simulink model "b6_pfc_rl"  (R2021b)
settings: Solver=FixedStepAuto  StartTime=0.0  StopTime=120.0  FixedStep=0.05  RelTol=1e-3
PreLoadFcn:
  | % Simulation parameters
  | %load exampleMap
  | 
  | % Lidar parameters
  | sensorOffset = [0,0];
  | scanAngles = linspace(-pi/2,pi/2,9)';
  | maxRange = 5;
InitFcn:
  | sampleTime = 0.05;
  | nMedianSize=3;
  | 
  | % Robot parameters
  | wheelRadius = 0.0335;
  | robotRadius = 0.116;
  | 
  | % Lidar parameters
  | sensorOffset = [0,0];
  | scanAngles = linspace(-pi/2,pi/2,9)';
  | maxRange = 5;
  | 
  | %%%%%%
  | ks=1;
  | c_ks=-1;
  | 
  | 
  | 
  | 
  | 
  | 
  | % Lidar parameters
  | sensorOffset = [0,0];
  | scanAngles = linspace(-pi/3,pi/3,20)';%y = linspace(x1,x2,n) 生成 n 个点。这些点的间距为 (x2-x1)/(n-1)。
  | maxRange = 0.4;
  | 
  | %%%%%%
  | ks=1;
  | 
  | 
  | 
  | 
  | 
  | A=0.3;
  | C=1.7;
  | B=(A+C)/2;
  | 
  | wp1=[A,A; B,A;  C,A; C,B;C,C; B,C; A,C;A,B];
  | bainjie2=[-0.5,-0.5;2.5,-0.5;-0.5,2.5;2.5,2.5;]
  | WAY_P=[wp1;wp1;wp1;wp1];
  | Target=[wp1;bainjie2];
  | 
  | %%%%%%%%%%%%%%%%%%%%%%%%%%%%%%%%%%%%%%%
  | Target_robot_4=[A  A]
  | Target_robot_5=[B  A]
  | Target_robot_6=[C  A]
  | 
  | Target_robot_1=[C  C]
  | Target_robot_2=[B  C]
  | Target_robot_3=[A  C]
  | 
  | 
  | %%%%%%%%%%%%%%%%%%%%%%%%%%%%%%%%%%%%
  | 
  | 
  | 
  | 
  | 
  | % paremeters of pure persuit
  | desired_v_robot_1=0.2
  | ... (+42 lines)
undefined symbols (not defined in the file or in its folder): Angular, DiscIntNeverNeededParam, Linear, Pose, Twist
libraries: robotlib x42, dspstat3 x18, mobileRoboticsLib x13, robotmobilelib x6, simulink x2, robotalgslib x1
(part 2 of 3)

== system b6_pfc_rl/controller/Ego Car 4 ==
  pose1 : Inport
  pose2 : Inport  Port=2
  leader_linear_vel : Inport  Port=3
  ego_linear_vel : Inport  Port=4
  ego_omega_vel : Inport  Port=5
  Delay : Delay  DelayLength=1  InitialCondition=0
  Signal Process : MATLAB Function  TreatAsAtomicUnit=on
  obs : Outport
  obs_flag : Outport  Port=2
  wires:
  pose1/1 -> Signal Process/1(pose1)
  Signal Process/1(observation) -> obs/1
  leader_linear_vel/1 -> Signal Process/3(leader_linear_vel)
  ego_omega_vel/1 -> Signal Process/5(ego_omega_vel), Delay/1
  pose2/1 -> Signal Process/2(pose2)
  ego_linear_vel/1 -> Signal Process/4(ego_linear_vel)
  Signal Process/2(obs_flag) -> obs_flag/1
  Delay/1 -> Signal Process/6(last_ego_omega_vel)

== system b6_pfc_rl/controller/Ego Car 5 ==
  pose1 : Inport
  pose2 : Inport  Port=2
  leader_linear_vel : Inport  Port=3
  ego_linear_vel : Inport  Port=4
  ego_omega_vel : Inport  Port=5
  Delay : Delay  DelayLength=1  InitialCondition=0
  Signal Process : MATLAB Function  TreatAsAtomicUnit=on
  obs : Outport
  obs_flag : Outport  Port=2
  wires:
  pose1/1 -> Signal Process/1(pose1)
  Signal Process/1(observation) -> obs/1
  leader_linear_vel/1 -> Signal Process/3(leader_linear_vel)
  ego_omega_vel/1 -> Signal Process/5(ego_omega_vel), Delay/1
  pose2/1 -> Signal Process/2(pose2)
  ego_linear_vel/1 -> Signal Process/4(ego_linear_vel)
  Signal Process/2(obs_flag) -> obs_flag/1
  Delay/1 -> Signal Process/6(last_ego_omega_vel)

== system b6_pfc_rl/controller/Subsystem1 ==
  WayPoints : Inport
  Pose : Inport  Port=2
  0 : Constant  Value=0
  1 : Constant  Value=0
  Adjust Velocities to Avoid Obstacles : Subsystem
  Compute Velocity and Heading for Path following : Subsystem
  Constant1 : Constant  Value=scanAngles
  Outputs1 : Subsystem
  v : Outport
  w : Outport  Port=2
  wires:
  Compute Velocity and Heading for Path following/3(W) -> Adjust Velocities to Avoid Obstacles/2(W), Outputs1/4(W)
  Pose/1 -> Compute Velocity and Heading for Path following/1(CurrentPose)
  Compute Velocity and Heading for Path following/2(V) -> Outputs1/3(V)
  WayPoints/1 -> Compute Velocity and Heading for Path following/2(Waypoints)
  1/1 -> Outputs1/5(CloseToGoal)
  Outputs1/1(v) -> v/1
  Outputs1/2(w) -> w/1
  Adjust Velocities to Avoid Obstacles/1(dW) -> Outputs1/2(dW)
  0/1 -> Outputs1/1(dV)
  Compute Velocity and Heading for Path following/1(TargetDir) -> Adjust Velocities to Avoid Obstacles/1(TargetDir)

== system b6_pfc_rl/controller/signal distribute ==
  In1 : Inport
  Demux5 : Demux  Outputs=12
  Mux{1,3..7} (6 alike) : Mux  Inputs=2
  Mux2 : Mux  Inputs=6
  Out1 : Outport
  wires:
  Mux7/1 -> Mux2/6
  Demux5/4 -> Mux3/2
  Mux1/1 -> Mux2/1
  Demux5/10 -> Mux6/2
  Demux5/7 -> Mux5/1
  Mux5/1 -> Mux2/4
  Mux3/1 -> Mux2/2
  Mux6/1 -> Mux2/5
  Mux4/1 -> Mux2/3
  Demux5/3 -> Mux3/1
  Demux5/8 -> Mux5/2
  Demux5/1 -> Mux1/1
  Demux5/9 -> Mux6/1
  Mux2/1 -> Out1/1
  Demux5/2 -> Mux1/2
  Demux5/11 -> Mux7/1
  Demux5/12 -> Mux7/2
  Demux5/5 -> Mux4/1
  Demux5/6 -> Mux4/2
  In1/1 -> Demux5/1

== system b6_pfc_rl/Subsystem/Car Pose Listener/Subsystem ==
  poseNew : Inport
  poseMsg : Inport  Port=2
  VW_New : Inport  Port=3
  VW_Msg : Inport  Port=4
  DiffSteer Kinematics : Subsystem
      settings: PortSchema="{\"entries\":[{\"content\":{\"sides\":[{\"content\":{\"connectorIds\":[\"In1\",\"In2\"]},\"type\":\"ConnectorPlacement.EquallySpacedRectSide\",\"uuid\":\"0032ed68-1de4-4b1c-b237-9372fedc8a7a\"},{\"content\":{\"connectorIds\":[\"Out1\",\"Out2\",\"Out3\"],\"side\":\"RIGHT\"},\"type\":\"ConnectorPlacement.EquallySpacedRectSide\",\"uuid\":\"d0c861bd-7497-47fe-b183-36da470ee2c6\"},{\"content\":{\"connectorIds\":[\"In3\",\"In4\"],\"side\":\"TOP\"},\"type\":\"ConnectorPlacement.EquallySpacedRectSide\",\"uuid\":\"5b685229-150b-4cb5-b33d-c61d28c4627e\"}]},\"type\":\"ConnectorPlacement.EquallySpacedConnector\",\"uuid\":\"4513c50b-5820-40cb-bb28-cc7c1b1322fe\"}],\"packageUris\":[\"http://schema.mathworks.com/mf0/Connector/R2020b\"],\"version\":\"1.0\"}"
  Median Filter : dspstat3/Median Filter  WindowLength=nMedianSize  SimulateUsing=Interpreted execution
      settings: SourceProductBaseCode=DS
  Median Filter1 : dspstat3/Median Filter  WindowLength=nMedianSize  SimulateUsing=Interpreted execution
      settings: SourceProductBaseCode=DS
  Median Filter2 : dspstat3/Median Filter  WindowLength=nMedianSize  SimulateUsing=Interpreted execution
      settings: SourceProductBaseCode=DS
  Mux7 : Mux  Inputs=3
  Sum : Sum  Inputs=++|
  Sum1 : Sum  Inputs=++|
  sensor2vCar : MATLAB Function  TreatAsAtomicUnit=on
  sensor2vCar4 : MATLAB Function  TreatAsAtomicUnit=on
  pose : Outport
  wires:
  Median Filter2/1 -> Mux7/3
  Median Filter1/1 -> Mux7/2
  Median Filter/1 -> Mux7/1
  sensor2vCar/4(flag) -> DiffSteer Kinematics/3(reset)
  DiffSteer Kinematics/2(y) -> Sum1/2
  sensor2vCar/3(yaw_init) -> DiffSteer Kinematics/4(yaw0)
  sensor2vCar/2(y_init) -> Sum1/1
  sensor2vCar/1(x_init) -> Sum/1
  DiffSteer Kinematics/1(x) -> Sum/2
  VW_New/1 -> sensor2vCar4/1(VW_New)
  Mux7/1 -> pose/1
  Sum/1 -> Median Filter/1
  DiffSteer Kinematics/3(psi) -> Median Filter2/1
  sensor2vCar4/1(V) -> DiffSteer Kinematics/1(u)
  Sum1/1 -> Median Filter1/1
  sensor2vCar4/2(W) -> DiffSteer Kinematics/2(w)
  poseNew/1 -> sensor2vCar/1(poseNew)
  poseMsg/1 -> sensor2vCar/2(poseMsg)
  VW_Msg/1 -> sensor2vCar4/2(VW_Msg)

== system b6_pfc_rl/Subsystem/Car Pose Listener1/Subsystem ==
  poseNew : Inport
  poseMsg : Inport  Port=2
  VW_New : Inport  Port=3
  VW_Msg : Inport  Port=4
  DiffSteer Kinematics : Subsystem
      settings: PortSchema="{\"entries\":[{\"content\":{\"sides\":[{\"content\":{\"connectorIds\":[\"In1\",\"In2\"]},\"type\":\"ConnectorPlacement.EquallySpacedRectSide\",\"uuid\":\"0032ed68-1de4-4b1c-b237-9372fedc8a7a\"},{\"content\":{\"connectorIds\":[\"Out1\",\"Out2\",\"Out3\"],\"side\":\"RIGHT\"},\"type\":\"ConnectorPlacement.EquallySpacedRectSide\",\"uuid\":\"d0c861bd-7497-47fe-b183-36da470ee2c6\"},{\"content\":{\"connectorIds\":[\"In3\",\"In4\"],\"side\":\"TOP\"},\"type\":\"ConnectorPlacement.EquallySpacedRectSide\",\"uuid\":\"5b685229-150b-4cb5-b33d-c61d28c4627e\"}]},\"type\":\"ConnectorPlacement.EquallySpacedConnector\",\"uuid\":\"4513c50b-5820-40cb-bb28-cc7c1b1322fe\"}],\"packageUris\":[\"http://schema.mathworks.com/mf0/Connector/R2020b\"],\"version\":\"1.0\"}"
  Median Filter : dspstat3/Median Filter  WindowLength=nMedianSize  SimulateUsing=Interpreted execution
      settings: SourceProductBaseCode=DS
  Median Filter1 : dspstat3/Median Filter  WindowLength=nMedianSize  SimulateUsing=Interpreted execution
      settings: SourceProductBaseCode=DS
  Median Filter2 : dspstat3/Median Filter  WindowLength=nMedianSize  SimulateUsing=Interpreted execution
      settings: SourceProductBaseCode=DS
  Mux7 : Mux  Inputs=3
  Sum : Sum  Inputs=++|
  Sum1 : Sum  Inputs=++|
  sensor2vCar : MATLAB Function  TreatAsAtomicUnit=on
  sensor2vCar4 : MATLAB Function  TreatAsAtomicUnit=on
  pose : Outport
  wires:
  Median Filter2/1 -> Mux7/3
  Median Filter1/1 -> Mux7/2
  Median Filter/1 -> Mux7/1
  sensor2vCar/4(flag) -> DiffSteer Kinematics/3(reset)
  DiffSteer Kinematics/2(y) -> Sum1/2
  sensor2vCar/3(yaw_init) -> DiffSteer Kinematics/4(yaw0)
  sensor2vCar/2(y_init) -> Sum1/1
  sensor2vCar/1(x_init) -> Sum/1
  DiffSteer Kinematics/1(x) -> Sum/2
  VW_New/1 -> sensor2vCar4/1(VW_New)
  Mux7/1 -> pose/1
  Sum/1 -> Median Filter/1
  DiffSteer Kinematics/3(psi) -> Median Filter2/1
  sensor2vCar4/1(V) -> DiffSteer Kinematics/1(u)
  Sum1/1 -> Median Filter1/1
  sensor2vCar4/2(W) -> DiffSteer Kinematics/2(w)
  poseNew/1 -> sensor2vCar/1(poseNew)
  poseMsg/1 -> sensor2vCar/2(poseMsg)
  VW_Msg/1 -> sensor2vCar4/2(VW_Msg)

== system b6_pfc_rl/Subsystem/Car Pose Listener2/Subsystem ==
  poseNew : Inport
  poseMsg : Inport  Port=2
  VW_New : Inport  Port=3
  VW_Msg : Inport  Port=4
  DiffSteer Kinematics : Subsystem
      settings: PortSchema="{\"entries\":[{\"content\":{\"sides\":[{\"content\":{\"connectorIds\":[\"In1\",\"In2\"]},\"type\":\"ConnectorPlacement.EquallySpacedRectSide\",\"uuid\":\"0032ed68-1de4-4b1c-b237-9372fedc8a7a\"},{\"content\":{\"connectorIds\":[\"Out1\",\"Out2\",\"Out3\"],\"side\":\"RIGHT\"},\"type\":\"ConnectorPlacement.EquallySpacedRectSide\",\"uuid\":\"d0c861bd-7497-47fe-b183-36da470ee2c6\"},{\"content\":{\"connectorIds\":[\"In3\",\"In4\"],\"side\":\"TOP\"},\"type\":\"ConnectorPlacement.EquallySpacedRectSide\",\"uuid\":\"5b685229-150b-4cb5-b33d-c61d28c4627e\"}]},\"type\":\"ConnectorPlacement.EquallySpacedConnector\",\"uuid\":\"4513c50b-5820-40cb-bb28-cc7c1b1322fe\"}],\"packageUris\":[\"http://schema.mathworks.com/mf0/Connector/R2020b\"],\"version\":\"1.0\"}"
  Median Filter : dspstat3/Median Filter  WindowLength=nMedianSize  SimulateUsing=Interpreted execution
      settings: SourceProductBaseCode=DS
  Median Filter1 : dspstat3/Median Filter  WindowLength=nMedianSize  SimulateUsing=Interpreted execution
      settings: SourceProductBaseCode=DS
  Median Filter2 : dspstat3/Median Filter  WindowLength=nMedianSize  SimulateUsing=Interpreted execution
      settings: SourceProductBaseCode=DS
  Mux7 : Mux  Inputs=3
  Sum : Sum  Inputs=++|
  Sum1 : Sum  Inputs=++|
  sensor2vCar : MATLAB Function  TreatAsAtomicUnit=on
  sensor2vCar4 : MATLAB Function  TreatAsAtomicUnit=on
  pose : Outport
  wires:
  Median Filter2/1 -> Mux7/3
  Median Filter1/1 -> Mux7/2
  Median Filter/1 -> Mux7/1
  sensor2vCar/4(flag) -> DiffSteer Kinematics/3(reset)
  DiffSteer Kinematics/2(y) -> Sum1/2
  sensor2vCar/3(yaw_init) -> DiffSteer Kinematics/4(yaw0)
  sensor2vCar/2(y_init) -> Sum1/1
  sensor2vCar/1(x_init) -> Sum/1
  DiffSteer Kinematics/1(x) -> Sum/2
  VW_New/1 -> sensor2vCar4/1(VW_New)
  Mux7/1 -> pose/1
  Sum/1 -> Median Filter/1
  DiffSteer Kinematics/3(psi) -> Median Filter2/1
  sensor2vCar4/1(V) -> DiffSteer Kinematics/1(u)
  Sum1/1 -> Median Filter1/1
  sensor2vCar4/2(W) -> DiffSteer Kinematics/2(w)
  poseNew/1 -> sensor2vCar/1(poseNew)
  poseMsg/1 -> sensor2vCar/2(poseMsg)
  VW_Msg/1 -> sensor2vCar4/2(VW_Msg)

== system b6_pfc_rl/Subsystem/Car Pose Listener3/Subsystem ==
  poseNew : Inport
  poseMsg : Inport  Port=2
  VW_New : Inport  Port=3
  VW_Msg : Inport  Port=4
  DiffSteer Kinematics : Subsystem
      settings: PortSchema="{\"entries\":[{\"content\":{\"sides\":[{\"content\":{\"connectorIds\":[\"In1\",\"In2\"]},\"type\":\"ConnectorPlacement.EquallySpacedRectSide\",\"uuid\":\"0032ed68-1de4-4b1c-b237-9372fedc8a7a\"},{\"content\":{\"connectorIds\":[\"Out1\",\"Out2\",\"Out3\"],\"side\":\"RIGHT\"},\"type\":\"ConnectorPlacement.EquallySpacedRectSide\",\"uuid\":\"d0c861bd-7497-47fe-b183-36da470ee2c6\"},{\"content\":{\"connectorIds\":[\"In3\",\"In4\"],\"side\":\"TOP\"},\"type\":\"ConnectorPlacement.EquallySpacedRectSide\",\"uuid\":\"5b685229-150b-4cb5-b33d-c61d28c4627e\"}]},\"type\":\"ConnectorPlacement.EquallySpacedConnector\",\"uuid\":\"4513c50b-5820-40cb-bb28-cc7c1b1322fe\"}],\"packageUris\":[\"http://schema.mathworks.com/mf0/Connector/R2020b\"],\"version\":\"1.0\"}"
  Median Filter : dspstat3/Median Filter  WindowLength=nMedianSize  SimulateUsing=Interpreted execution
      settings: SourceProductBaseCode=DS
  Median Filter1 : dspstat3/Median Filter  WindowLength=nMedianSize  SimulateUsing=Interpreted execution
      settings: SourceProductBaseCode=DS
  Median Filter2 : dspstat3/Median Filter  WindowLength=nMedianSize  SimulateUsing=Interpreted execution
      settings: SourceProductBaseCode=DS
  Mux7 : Mux  Inputs=3
  Sum : Sum  Inputs=++|
  Sum1 : Sum  Inputs=++|
  sensor2vCar : MATLAB Function  TreatAsAtomicUnit=on
  sensor2vCar4 : MATLAB Function  TreatAsAtomicUnit=on
  pose : Outport
  wires:
  Median Filter2/1 -> Mux7/3
  Median Filter1/1 -> Mux7/2
  Median Filter/1 -> Mux7/1
  sensor2vCar/4(flag) -> DiffSteer Kinematics/3(reset)
  DiffSteer Kinematics/2(y) -> Sum1/2
  sensor2vCar/3(yaw_init) -> DiffSteer Kinematics/4(yaw0)
  sensor2vCar/2(y_init) -> Sum1/1
  sensor2vCar/1(x_init) -> Sum/1
  DiffSteer Kinematics/1(x) -> Sum/2
  VW_New/1 -> sensor2vCar4/1(VW_New)
  Mux7/1 -> pose/1
  Sum/1 -> Median Filter/1
  DiffSteer Kinematics/3(psi) -> Median Filter2/1
  sensor2vCar4/1(V) -> DiffSteer Kinematics/1(u)
  Sum1/1 -> Median Filter1/1
  sensor2vCar4/2(W) -> DiffSteer Kinematics/2(w)
  poseNew/1 -> sensor2vCar/1(poseNew)
  poseMsg/1 -> sensor2vCar/2(poseMsg)
  VW_Msg/1 -> sensor2vCar4/2(VW_Msg)

== system b6_pfc_rl/Subsystem/Car Pose Listener4/Subsystem ==
  poseNew : Inport
  poseMsg : Inport  Port=2
  VW_New : Inport  Port=3
  VW_Msg : Inport  Port=4
  DiffSteer Kinematics : Subsystem
      settings: PortSchema="{\"entries\":[{\"content\":{\"sides\":[{\"content\":{\"connectorIds\":[\"In1\",\"In2\"]},\"type\":\"ConnectorPlacement.EquallySpacedRectSide\",\"uuid\":\"0032ed68-1de4-4b1c-b237-9372fedc8a7a\"},{\"content\":{\"connectorIds\":[\"Out1\",\"Out2\",\"Out3\"],\"side\":\"RIGHT\"},\"type\":\"ConnectorPlacement.EquallySpacedRectSide\",\"uuid\":\"d0c861bd-7497-47fe-b183-36da470ee2c6\"},{\"content\":{\"connectorIds\":[\"In3\",\"In4\"],\"side\":\"TOP\"},\"type\":\"ConnectorPlacement.EquallySpacedRectSide\",\"uuid\":\"5b685229-150b-4cb5-b33d-c61d28c4627e\"}]},\"type\":\"ConnectorPlacement.EquallySpacedConnector\",\"uuid\":\"4513c50b-5820-40cb-bb28-cc7c1b1322fe\"}],\"packageUris\":[\"http://schema.mathworks.com/mf0/Connector/R2020b\"],\"version\":\"1.0\"}"
  Median Filter : dspstat3/Median Filter  WindowLength=nMedianSize  SimulateUsing=Interpreted execution
      settings: SourceProductBaseCode=DS
  Median Filter1 : dspstat3/Median Filter  WindowLength=nMedianSize  SimulateUsing=Interpreted execution
      settings: SourceProductBaseCode=DS
  Median Filter2 : dspstat3/Median Filter  WindowLength=nMedianSize  SimulateUsing=Interpreted execution
      settings: SourceProductBaseCode=DS
  Mux7 : Mux  Inputs=3
  Sum : Sum  Inputs=++|
  Sum1 : Sum  Inputs=++|
  sensor2vCar : MATLAB Function  TreatAsAtomicUnit=on
  sensor2vCar4 : MATLAB Function  TreatAsAtomicUnit=on
  pose : Outport
  wires:
  Median Filter2/1 -> Mux7/3
  Median Filter1/1 -> Mux7/2
  Median Filter/1 -> Mux7/1
  sensor2vCar/4(flag) -> DiffSteer Kinematics/3(reset)
  DiffSteer Kinematics/2(y) -> Sum1/2
  sensor2vCar/3(yaw_init) -> DiffSteer Kinematics/4(yaw0)
  sensor2vCar/2(y_init) -> Sum1/1
  sensor2vCar/1(x_init) -> Sum/1
  DiffSteer Kinematics/1(x) -> Sum/2
  VW_New/1 -> sensor2vCar4/1(VW_New)
  Mux7/1 -> pose/1
  Sum/1 -> Median Filter/1
  DiffSteer Kinematics/3(psi) -> Median Filter2/1
  sensor2vCar4/1(V) -> DiffSteer Kinematics/1(u)
  Sum1/1 -> Median Filter1/1
  sensor2vCar4/2(W) -> DiffSteer Kinematics/2(w)
  poseNew/1 -> sensor2vCar/1(poseNew)
  poseMsg/1 -> sensor2vCar/2(poseMsg)
  VW_Msg/1 -> sensor2vCar4/2(VW_Msg)

== system b6_pfc_rl/Subsystem/Car Pose Listener5/Subsystem ==
  poseNew : Inport
  poseMsg : Inport  Port=2
  VW_New : Inport  Port=3
  VW_Msg : Inport  Port=4
  DiffSteer Kinematics : Subsystem
      settings: PortSchema="{\"entries\":[{\"content\":{\"sides\":[{\"content\":{\"connectorIds\":[\"In1\",\"In2\"]},\"type\":\"ConnectorPlacement.EquallySpacedRectSide\",\"uuid\":\"0032ed68-1de4-4b1c-b237-9372fedc8a7a\"},{\"content\":{\"connectorIds\":[\"Out1\",\"Out2\",\"Out3\"],\"side\":\"RIGHT\"},\"type\":\"ConnectorPlacement.EquallySpacedRectSide\",\"uuid\":\"d0c861bd-7497-47fe-b183-36da470ee2c6\"},{\"content\":{\"connectorIds\":[\"In3\",\"In4\"],\"side\":\"TOP\"},\"type\":\"ConnectorPlacement.EquallySpacedRectSide\",\"uuid\":\"5b685229-150b-4cb5-b33d-c61d28c4627e\"}]},\"type\":\"ConnectorPlacement.EquallySpacedConnector\",\"uuid\":\"4513c50b-5820-40cb-bb28-cc7c1b1322fe\"}],\"packageUris\":[\"http://schema.mathworks.com/mf0/Connector/R2020b\"],\"version\":\"1.0\"}"
  Median Filter : dspstat3/Median Filter  WindowLength=nMedianSize  SimulateUsing=Interpreted execution
      settings: SourceProductBaseCode=DS
  Median Filter1 : dspstat3/Median Filter  WindowLength=nMedianSize  SimulateUsing=Interpreted execution
      settings: SourceProductBaseCode=DS
  Median Filter2 : dspstat3/Median Filter  WindowLength=nMedianSize  SimulateUsing=Interpreted execution
      settings: SourceProductBaseCode=DS
  Mux7 : Mux  Inputs=3
  Sum : Sum  Inputs=++|
  Sum1 : Sum  Inputs=++|
  sensor2vCar : MATLAB Function  TreatAsAtomicUnit=on
  sensor2vCar4 : MATLAB Function  TreatAsAtomicUnit=on
  pose : Outport
  wires:
  Median Filter2/1 -> Mux7/3
  Median Filter1/1 -> Mux7/2
  Median Filter/1 -> Mux7/1
  sensor2vCar/4(flag) -> DiffSteer Kinematics/3(reset)
  DiffSteer Kinematics/2(y) -> Sum1/2
  sensor2vCar/3(yaw_init) -> DiffSteer Kinematics/4(yaw0)
  sensor2vCar/2(y_init) -> Sum1/1
  sensor2vCar/1(x_init) -> Sum/1
  DiffSteer Kinematics/1(x) -> Sum/2
  VW_New/1 -> sensor2vCar4/1(VW_New)
  Mux7/1 -> pose/1
  Sum/1 -> Median Filter/1
  DiffSteer Kinematics/3(psi) -> Median Filter2/1
  sensor2vCar4/1(V) -> DiffSteer Kinematics/1(u)
  Sum1/1 -> Median Filter1/1
  sensor2vCar4/2(W) -> DiffSteer Kinematics/2(w)
  poseNew/1 -> sensor2vCar/1(poseNew)
  poseMsg/1 -> sensor2vCar/2(poseMsg)
  VW_Msg/1 -> sensor2vCar4/2(VW_Msg)

== system b6_pfc_rl/controller/Subsystem1/Adjust Velocities to Avoid Obstacles ==
  TargetDir : Inport
  W : Inport  Port=2
  Path Following : Subsystem  TreatAsAtomicUnit=on
  dW : Outport  VectorParamsAs1DForOutWhenUnconnected=off
  wires:
  Path Following/1(dW) -> dW/1
  W/1 -> Path Following/2(AngularVelocity)
  TargetDir/1 -> Path Following/1(SteeringDirection)

== system b6_pfc_rl/controller/Subsystem1/Compute Velocity and Heading for Path following ==
  note: Check If Close To Goal
  CurrentPose : Inport
  Waypoints : Inport  Port=2
  " Extract Goal" : MATLAB Function  TreatAsAtomicUnit=on
  Dot Product : DotProduct  InputSameDT=on  OutDataTypeStr=Inherit: Inherit via internal rule
  GoalRadius : Constant  Value=0.1
  Pure Pursuit : robotalgslib/Pure Pursuit  DesiredLinearVelocity=desired_v_robot_1  MaxAngularVelocity=desired_w_robot_1  LookaheadDistance=desired_lookahead_robot_1  TargetDirPort=on  SimulateUsing=Code generation
  Relational Operator : RelationalOperator  Operator=<=  OutDataTypeStr=boolean  RndMeth=Simplest
  Selector : Selector  InputPortWidth=3  IndexOptions=Index vector (dialog)  Indices=[1 2]  OutputSizes=1
  Sqrt : Sqrt  SaturateOnIntegerOverflow=on
  Subtract : Sum  Inputs=+-
  TargetDir : Outport  VectorParamsAs1DForOutWhenUnconnected=off
  V : Outport  Port=2  VectorParamsAs1DForOutWhenUnconnected=off
  W : Outport  Port=3  VectorParamsAs1DForOutWhenUnconnected=off
  CloseToGoal : Outport  Port=4  VectorParamsAs1DForOutWhenUnconnected=off
  wires:
  Pure Pursuit/3 -> TargetDir/1
  Pure Pursuit/2 -> W/1
  Pure Pursuit/1 -> V/1
  " Extract Goal"/1(Goal) -> Subtract/2
  Waypoints/1 -> " Extract Goal"/1(Waypoints), Pure Pursuit/2
  CurrentPose/1 -> Selector/1, Pure Pursuit/1
  Relational Operator/1 -> CloseToGoal/1
  GoalRadius/1 -> Relational Operator/2
  Selector/1 -> Subtract/1
  Dot Product/1 -> Sqrt/1
  Sqrt/1 -> Relational Operator/1
  Subtract/1 -> Dot Product/1, Dot Product/2

== system b6_pfc_rl/controller/Subsystem1/Outputs1 ==
  dV : Inport
  dW : Inport  Port=2
  V : Inport  Port=3
  W : Inport  Port=4
  CloseToGoal : Inport  Port=5
  Add : Sum
  Add1 : Sum
  Logical Operator : Logic  Operator=NOT  AllPortsSameDT=off  OutDataTypeStr=boolean
  Product : Product
  Product1 : Product
  v : Outport
  w : Outport  Port=2
  wires:
  V/1 -> Add/2
  W/1 -> Add1/2
  dV/1 -> Add/1
  dW/1 -> Add1/1
  CloseToGoal/1 -> Logical Operator/1
  Add/1 -> Product/1
  Add1/1 -> Product1/1
  Product1/1 -> w/1
  Product/1 -> v/1
  Logical Operator/1 -> Product1/2, Product/2

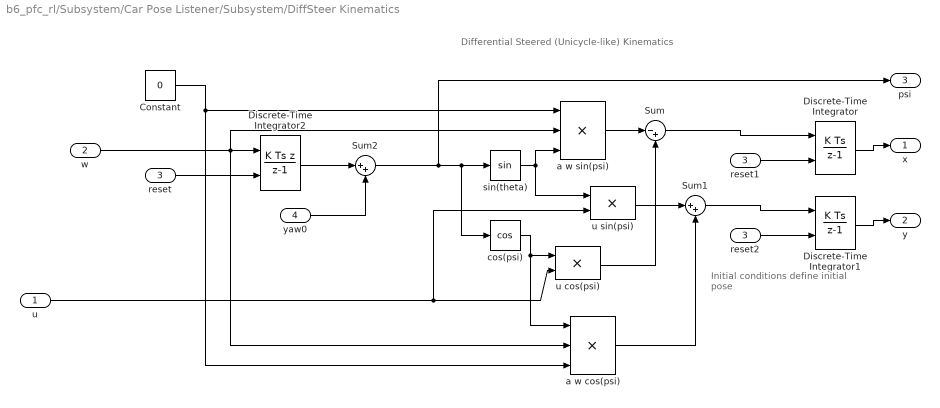
== system b6_pfc_rl/Subsystem/Car Pose Listener/Subsystem/DiffSteer Kinematics ==
  note: Initial conditions define
      | initial pose
  note: Differential Steered (Unicycle-like) Kinematics
  u : Inport
  w : Inport  Port=2
  reset : Inport  Port=3
  yaw0 : Inport  Port=4
  Constant : Constant  Value=0
  Discrete-Time Integrator : DiscreteIntegrator  ExternalReset=falling  SampleTime=-1  ICPrevOutput=DiscIntNeverNeededParam  ICPrevScaledInput=DiscIntNeverNeededParam
  Discrete-Time Integrator1 : DiscreteIntegrator  ExternalReset=falling  SampleTime=-1  ICPrevOutput=DiscIntNeverNeededParam  ICPrevScaledInput=DiscIntNeverNeededParam
  Discrete-Time Integrator2 : DiscreteIntegrator  IntegratorMethod=Integration: Backward Euler  ExternalReset=falling  SampleTime=-1  ICPrevOutput=DiscIntNeverNeededParam  ICPrevScaledInput=DiscIntNeverNeededParam
  Sum : Sum  Inputs=|-+  SaturateOnIntegerOverflow=on
  Sum1 : Sum  Inputs=|++  SaturateOnIntegerOverflow=on
  Sum2 : Sum  Inputs=|++
  a w cos(psi) : Product  Inputs=3  SaturateOnIntegerOverflow=on  OutDataTypeStr=Inherit: Same as first input
  a w sin(psi) : Product  Inputs=3  SaturateOnIntegerOverflow=on  OutDataTypeStr=Inherit: Same as first input
  cos(psi) : Trigonometry  Operator=cos
  reset1 : InportShadow  Port=3
  reset2 : InportShadow  Port=3
  sin(theta) : Trigonometry
  u cos(psi) : Product  SaturateOnIntegerOverflow=on  OutDataTypeStr=Inherit: Same as first input
  u sin(psi) : Product  SaturateOnIntegerOverflow=on  OutDataTypeStr=Inherit: Same as first input
  x : Outport
  y : Outport  Port=2
  psi : Outport  Port=3
  wires:
  yaw0/1 -> Sum2/2
  reset2/1 -> Discrete-Time Integrator1/2
  reset1/1 -> Discrete-Time Integrator/2
  reset/1 -> Discrete-Time Integrator2/2
  u sin(psi)/1 -> Sum1/1
  cos(psi)/1 -> u cos(psi)/1, a w cos(psi)/1
  w/1 -> a w cos(psi)/2, a w sin(psi)/2, Discrete-Time Integrator2/1
  Constant/1 -> a w sin(psi)/1, a w cos(psi)/3
  Discrete-Time Integrator/1 -> x/1
  Sum/1 -> Discrete-Time Integrator/1
  sin(theta)/1 -> a w sin(psi)/3, u sin(psi)/1
  a w cos(psi)/1 -> Sum1/2
  Sum2/1 -> psi/1, sin(theta)/1, cos(psi)/1
  u cos(psi)/1 -> Sum/2
  u/1 -> u sin(psi)/2, u cos(psi)/2
  a w sin(psi)/1 -> Sum/1
  Sum1/1 -> Discrete-Time Integrator1/1
  Discrete-Time Integrator1/1 -> y/1
  Discrete-Time Integrator2/1 -> Sum2/1

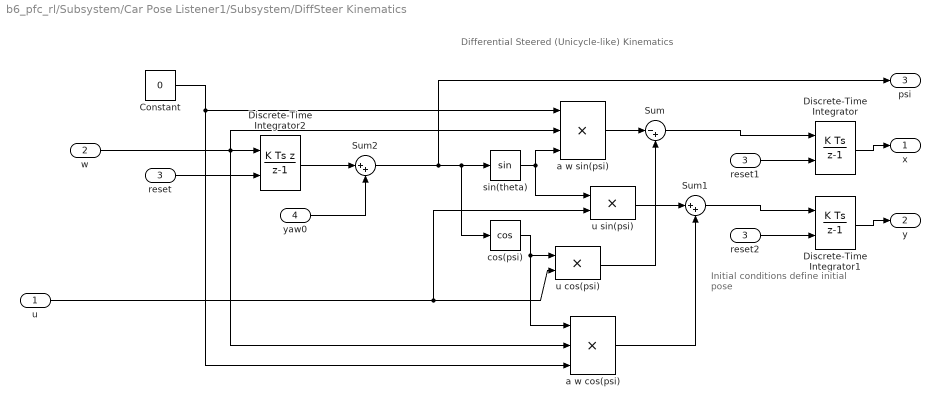
== system b6_pfc_rl/Subsystem/Car Pose Listener1/Subsystem/DiffSteer Kinematics ==
  note: Initial conditions define
      | initial pose
  note: Differential Steered (Unicycle-like) Kinematics
  u : Inport
  w : Inport  Port=2
  reset : Inport  Port=3
  yaw0 : Inport  Port=4
  Constant : Constant  Value=0
  Discrete-Time Integrator : DiscreteIntegrator  ExternalReset=falling  SampleTime=-1  ICPrevOutput=DiscIntNeverNeededParam  ICPrevScaledInput=DiscIntNeverNeededParam
  Discrete-Time Integrator1 : DiscreteIntegrator  ExternalReset=falling  SampleTime=-1  ICPrevOutput=DiscIntNeverNeededParam  ICPrevScaledInput=DiscIntNeverNeededParam
  Discrete-Time Integrator2 : DiscreteIntegrator  IntegratorMethod=Integration: Backward Euler  ExternalReset=falling  SampleTime=-1  ICPrevOutput=DiscIntNeverNeededParam  ICPrevScaledInput=DiscIntNeverNeededParam
  Sum : Sum  Inputs=|-+  SaturateOnIntegerOverflow=on
  Sum1 : Sum  Inputs=|++  SaturateOnIntegerOverflow=on
  Sum2 : Sum  Inputs=|++
  a w cos(psi) : Product  Inputs=3  SaturateOnIntegerOverflow=on  OutDataTypeStr=Inherit: Same as first input
  a w sin(psi) : Product  Inputs=3  SaturateOnIntegerOverflow=on  OutDataTypeStr=Inherit: Same as first input
  cos(psi) : Trigonometry  Operator=cos
  reset1 : InportShadow  Port=3
  reset2 : InportShadow  Port=3
  sin(theta) : Trigonometry
  u cos(psi) : Product  SaturateOnIntegerOverflow=on  OutDataTypeStr=Inherit: Same as first input
  u sin(psi) : Product  SaturateOnIntegerOverflow=on  OutDataTypeStr=Inherit: Same as first input
  x : Outport
  y : Outport  Port=2
  psi : Outport  Port=3
  wires:
  yaw0/1 -> Sum2/2
  reset2/1 -> Discrete-Time Integrator1/2
  reset1/1 -> Discrete-Time Integrator/2
  reset/1 -> Discrete-Time Integrator2/2
  u sin(psi)/1 -> Sum1/1
  cos(psi)/1 -> u cos(psi)/1, a w cos(psi)/1
  w/1 -> a w cos(psi)/2, a w sin(psi)/2, Discrete-Time Integrator2/1
  Constant/1 -> a w sin(psi)/1, a w cos(psi)/3
  Discrete-Time Integrator/1 -> x/1
  Sum/1 -> Discrete-Time Integrator/1
  sin(theta)/1 -> a w sin(psi)/3, u sin(psi)/1
  a w cos(psi)/1 -> Sum1/2
  Sum2/1 -> psi/1, sin(theta)/1, cos(psi)/1
  u cos(psi)/1 -> Sum/2
  u/1 -> u sin(psi)/2, u cos(psi)/2
  a w sin(psi)/1 -> Sum/1
  Sum1/1 -> Discrete-Time Integrator1/1
  Discrete-Time Integrator1/1 -> y/1
  Discrete-Time Integrator2/1 -> Sum2/1

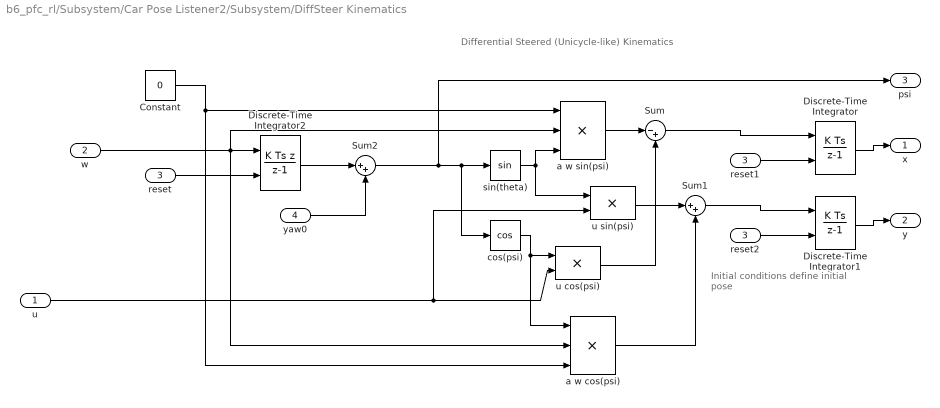
== system b6_pfc_rl/Subsystem/Car Pose Listener2/Subsystem/DiffSteer Kinematics ==
  note: Initial conditions define
      | initial pose
  note: Differential Steered (Unicycle-like) Kinematics
  u : Inport
  w : Inport  Port=2
  reset : Inport  Port=3
  yaw0 : Inport  Port=4
  Constant : Constant  Value=0
  Discrete-Time Integrator : DiscreteIntegrator  ExternalReset=falling  SampleTime=-1  ICPrevOutput=DiscIntNeverNeededParam  ICPrevScaledInput=DiscIntNeverNeededParam
  Discrete-Time Integrator1 : DiscreteIntegrator  ExternalReset=falling  SampleTime=-1  ICPrevOutput=DiscIntNeverNeededParam  ICPrevScaledInput=DiscIntNeverNeededParam
  Discrete-Time Integrator2 : DiscreteIntegrator  IntegratorMethod=Integration: Backward Euler  ExternalReset=falling  SampleTime=-1  ICPrevOutput=DiscIntNeverNeededParam  ICPrevScaledInput=DiscIntNeverNeededParam
  Sum : Sum  Inputs=|-+  SaturateOnIntegerOverflow=on
  Sum1 : Sum  Inputs=|++  SaturateOnIntegerOverflow=on
  Sum2 : Sum  Inputs=|++
  a w cos(psi) : Product  Inputs=3  SaturateOnIntegerOverflow=on  OutDataTypeStr=Inherit: Same as first input
  a w sin(psi) : Product  Inputs=3  SaturateOnIntegerOverflow=on  OutDataTypeStr=Inherit: Same as first input
  cos(psi) : Trigonometry  Operator=cos
  reset1 : InportShadow  Port=3
  reset2 : InportShadow  Port=3
  sin(theta) : Trigonometry
  u cos(psi) : Product  SaturateOnIntegerOverflow=on  OutDataTypeStr=Inherit: Same as first input
  u sin(psi) : Product  SaturateOnIntegerOverflow=on  OutDataTypeStr=Inherit: Same as first input
  x : Outport
  y : Outport  Port=2
  psi : Outport  Port=3
  wires:
  yaw0/1 -> Sum2/2
  reset2/1 -> Discrete-Time Integrator1/2
  reset1/1 -> Discrete-Time Integrator/2
  reset/1 -> Discrete-Time Integrator2/2
  u sin(psi)/1 -> Sum1/1
  cos(psi)/1 -> u cos(psi)/1, a w cos(psi)/1
  w/1 -> a w cos(psi)/2, a w sin(psi)/2, Discrete-Time Integrator2/1
  Constant/1 -> a w sin(psi)/1, a w cos(psi)/3
  Discrete-Time Integrator/1 -> x/1
  Sum/1 -> Discrete-Time Integrator/1
  sin(theta)/1 -> a w sin(psi)/3, u sin(psi)/1
  a w cos(psi)/1 -> Sum1/2
  Sum2/1 -> psi/1, sin(theta)/1, cos(psi)/1
  u cos(psi)/1 -> Sum/2
  u/1 -> u sin(psi)/2, u cos(psi)/2
  a w sin(psi)/1 -> Sum/1
  Sum1/1 -> Discrete-Time Integrator1/1
  Discrete-Time Integrator1/1 -> y/1
  Discrete-Time Integrator2/1 -> Sum2/1

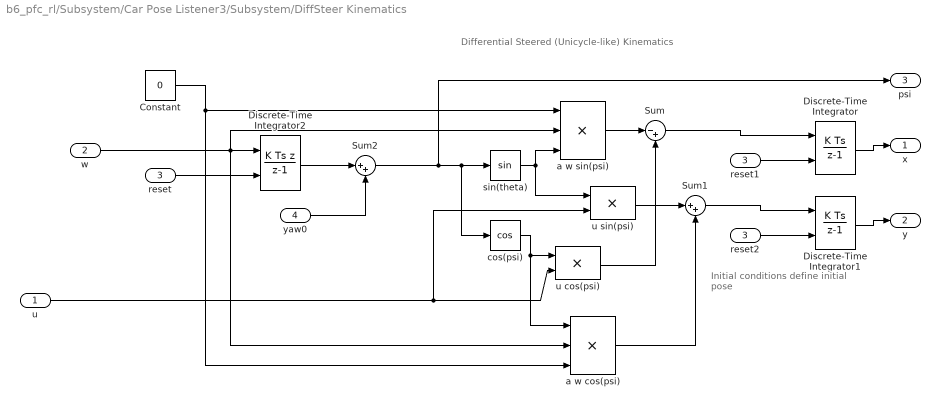
== system b6_pfc_rl/Subsystem/Car Pose Listener3/Subsystem/DiffSteer Kinematics ==
  note: Initial conditions define
      | initial pose
  note: Differential Steered (Unicycle-like) Kinematics
  u : Inport
  w : Inport  Port=2
  reset : Inport  Port=3
  yaw0 : Inport  Port=4
  Constant : Constant  Value=0
  Discrete-Time Integrator : DiscreteIntegrator  ExternalReset=falling  SampleTime=-1  ICPrevOutput=DiscIntNeverNeededParam  ICPrevScaledInput=DiscIntNeverNeededParam
  Discrete-Time Integrator1 : DiscreteIntegrator  ExternalReset=falling  SampleTime=-1  ICPrevOutput=DiscIntNeverNeededParam  ICPrevScaledInput=DiscIntNeverNeededParam
  Discrete-Time Integrator2 : DiscreteIntegrator  IntegratorMethod=Integration: Backward Euler  ExternalReset=falling  SampleTime=-1  ICPrevOutput=DiscIntNeverNeededParam  ICPrevScaledInput=DiscIntNeverNeededParam
  Sum : Sum  Inputs=|-+  SaturateOnIntegerOverflow=on
  Sum1 : Sum  Inputs=|++  SaturateOnIntegerOverflow=on
  Sum2 : Sum  Inputs=|++
  a w cos(psi) : Product  Inputs=3  SaturateOnIntegerOverflow=on  OutDataTypeStr=Inherit: Same as first input
  a w sin(psi) : Product  Inputs=3  SaturateOnIntegerOverflow=on  OutDataTypeStr=Inherit: Same as first input
  cos(psi) : Trigonometry  Operator=cos
  reset1 : InportShadow  Port=3
  reset2 : InportShadow  Port=3
  sin(theta) : Trigonometry
  u cos(psi) : Product  SaturateOnIntegerOverflow=on  OutDataTypeStr=Inherit: Same as first input
  u sin(psi) : Product  SaturateOnIntegerOverflow=on  OutDataTypeStr=Inherit: Same as first input
  x : Outport
  y : Outport  Port=2
  psi : Outport  Port=3
  wires:
  yaw0/1 -> Sum2/2
  reset2/1 -> Discrete-Time Integrator1/2
  reset1/1 -> Discrete-Time Integrator/2
  reset/1 -> Discrete-Time Integrator2/2
  u sin(psi)/1 -> Sum1/1
  cos(psi)/1 -> u cos(psi)/1, a w cos(psi)/1
  w/1 -> a w cos(psi)/2, a w sin(psi)/2, Discrete-Time Integrator2/1
  Constant/1 -> a w sin(psi)/1, a w cos(psi)/3
  Discrete-Time Integrator/1 -> x/1
  Sum/1 -> Discrete-Time Integrator/1
  sin(theta)/1 -> a w sin(psi)/3, u sin(psi)/1
  a w cos(psi)/1 -> Sum1/2
  Sum2/1 -> psi/1, sin(theta)/1, cos(psi)/1
  u cos(psi)/1 -> Sum/2
  u/1 -> u sin(psi)/2, u cos(psi)/2
  a w sin(psi)/1 -> Sum/1
  Sum1/1 -> Discrete-Time Integrator1/1
  Discrete-Time Integrator1/1 -> y/1
  Discrete-Time Integrator2/1 -> Sum2/1

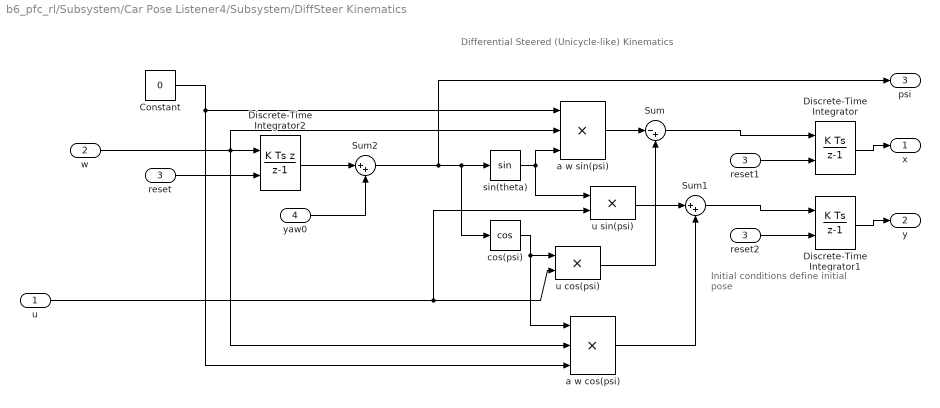
== system b6_pfc_rl/Subsystem/Car Pose Listener4/Subsystem/DiffSteer Kinematics ==
  note: Initial conditions define
      | initial pose
  note: Differential Steered (Unicycle-like) Kinematics
  u : Inport
  w : Inport  Port=2
  reset : Inport  Port=3
  yaw0 : Inport  Port=4
  Constant : Constant  Value=0
  Discrete-Time Integrator : DiscreteIntegrator  ExternalReset=falling  SampleTime=-1  ICPrevOutput=DiscIntNeverNeededParam  ICPrevScaledInput=DiscIntNeverNeededParam
  Discrete-Time Integrator1 : DiscreteIntegrator  ExternalReset=falling  SampleTime=-1  ICPrevOutput=DiscIntNeverNeededParam  ICPrevScaledInput=DiscIntNeverNeededParam
  Discrete-Time Integrator2 : DiscreteIntegrator  IntegratorMethod=Integration: Backward Euler  ExternalReset=falling  SampleTime=-1  ICPrevOutput=DiscIntNeverNeededParam  ICPrevScaledInput=DiscIntNeverNeededParam
  Sum : Sum  Inputs=|-+  SaturateOnIntegerOverflow=on
  Sum1 : Sum  Inputs=|++  SaturateOnIntegerOverflow=on
  Sum2 : Sum  Inputs=|++
  a w cos(psi) : Product  Inputs=3  SaturateOnIntegerOverflow=on  OutDataTypeStr=Inherit: Same as first input
  a w sin(psi) : Product  Inputs=3  SaturateOnIntegerOverflow=on  OutDataTypeStr=Inherit: Same as first input
  cos(psi) : Trigonometry  Operator=cos
  reset1 : InportShadow  Port=3
  reset2 : InportShadow  Port=3
  sin(theta) : Trigonometry
  u cos(psi) : Product  SaturateOnIntegerOverflow=on  OutDataTypeStr=Inherit: Same as first input
  u sin(psi) : Product  SaturateOnIntegerOverflow=on  OutDataTypeStr=Inherit: Same as first input
  x : Outport
  y : Outport  Port=2
  psi : Outport  Port=3
  wires:
  yaw0/1 -> Sum2/2
  reset2/1 -> Discrete-Time Integrator1/2
  reset1/1 -> Discrete-Time Integrator/2
  reset/1 -> Discrete-Time Integrator2/2
  u sin(psi)/1 -> Sum1/1
  cos(psi)/1 -> u cos(psi)/1, a w cos(psi)/1
  w/1 -> a w cos(psi)/2, a w sin(psi)/2, Discrete-Time Integrator2/1
  Constant/1 -> a w sin(psi)/1, a w cos(psi)/3
  Discrete-Time Integrator/1 -> x/1
  Sum/1 -> Discrete-Time Integrator/1
  sin(theta)/1 -> a w sin(psi)/3, u sin(psi)/1
  a w cos(psi)/1 -> Sum1/2
  Sum2/1 -> psi/1, sin(theta)/1, cos(psi)/1
  u cos(psi)/1 -> Sum/2
  u/1 -> u sin(psi)/2, u cos(psi)/2
  a w sin(psi)/1 -> Sum/1
  Sum1/1 -> Discrete-Time Integrator1/1
  Discrete-Time Integrator1/1 -> y/1
  Discrete-Time Integrator2/1 -> Sum2/1

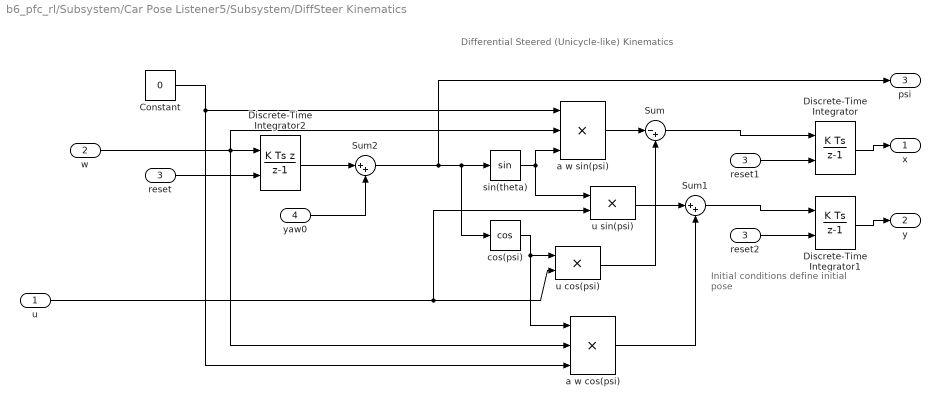
== system b6_pfc_rl/Subsystem/Car Pose Listener5/Subsystem/DiffSteer Kinematics ==
  note: Initial conditions define
      | initial pose
  note: Differential Steered (Unicycle-like) Kinematics
  u : Inport
  w : Inport  Port=2
  reset : Inport  Port=3
  yaw0 : Inport  Port=4
  Constant : Constant  Value=0
  Discrete-Time Integrator : DiscreteIntegrator  ExternalReset=falling  SampleTime=-1  ICPrevOutput=DiscIntNeverNeededParam  ICPrevScaledInput=DiscIntNeverNeededParam
  Discrete-Time Integrator1 : DiscreteIntegrator  ExternalReset=falling  SampleTime=-1  ICPrevOutput=DiscIntNeverNeededParam  ICPrevScaledInput=DiscIntNeverNeededParam
  Discrete-Time Integrator2 : DiscreteIntegrator  IntegratorMethod=Integration: Backward Euler  ExternalReset=falling  SampleTime=-1  ICPrevOutput=DiscIntNeverNeededParam  ICPrevScaledInput=DiscIntNeverNeededParam
  Sum : Sum  Inputs=|-+  SaturateOnIntegerOverflow=on
  Sum1 : Sum  Inputs=|++  SaturateOnIntegerOverflow=on
  Sum2 : Sum  Inputs=|++
  a w cos(psi) : Product  Inputs=3  SaturateOnIntegerOverflow=on  OutDataTypeStr=Inherit: Same as first input
  a w sin(psi) : Product  Inputs=3  SaturateOnIntegerOverflow=on  OutDataTypeStr=Inherit: Same as first input
  cos(psi) : Trigonometry  Operator=cos
  reset1 : InportShadow  Port=3
  reset2 : InportShadow  Port=3
  sin(theta) : Trigonometry
  u cos(psi) : Product  SaturateOnIntegerOverflow=on  OutDataTypeStr=Inherit: Same as first input
  u sin(psi) : Product  SaturateOnIntegerOverflow=on  OutDataTypeStr=Inherit: Same as first input
  x : Outport
  y : Outport  Port=2
  psi : Outport  Port=3
  wires:
  yaw0/1 -> Sum2/2
  reset2/1 -> Discrete-Time Integrator1/2
  reset1/1 -> Discrete-Time Integrator/2
  reset/1 -> Discrete-Time Integrator2/2
  u sin(psi)/1 -> Sum1/1
  cos(psi)/1 -> u cos(psi)/1, a w cos(psi)/1
  w/1 -> a w cos(psi)/2, a w sin(psi)/2, Discrete-Time Integrator2/1
  Constant/1 -> a w sin(psi)/1, a w cos(psi)/3
  Discrete-Time Integrator/1 -> x/1
  Sum/1 -> Discrete-Time Integrator/1
  sin(theta)/1 -> a w sin(psi)/3, u sin(psi)/1
  a w cos(psi)/1 -> Sum1/2
  Sum2/1 -> psi/1, sin(theta)/1, cos(psi)/1
  u cos(psi)/1 -> Sum/2
  u/1 -> u sin(psi)/2, u cos(psi)/2
  a w sin(psi)/1 -> Sum/1
  Sum1/1 -> Discrete-Time Integrator1/1
  Discrete-Time Integrator1/1 -> y/1
  Discrete-Time Integrator2/1 -> Sum2/1

== system b6_pfc_rl/controller/Subsystem1/Adjust Velocities to Avoid Obstacles/Path Following ==
  SteeringDirection : Inport
  AngularVelocity : Inport  Port=2
  Compute Angular Velocity : MATLAB Function  TreatAsAtomicUnit=on
  MaxAngularVelocity : Constant
  Subtract : Sum  Inputs=+-
  dW : Outport  VectorParamsAs1DForOutWhenUnconnected=off
  wires:
  MaxAngularVelocity/1 -> Compute Angular Velocity/2(wMax)
  SteeringDirection/1 -> Compute Angular Velocity/1(steeringDir)
  Subtract/1 -> dW/1
  Compute Angular Velocity/1(w) -> Subtract/1
  AngularVelocity/1 -> Subtract/2

== matlab function b6_pfc_rl/ROS_simulation/ros1/MATLAB Function3 ==
  data: IsNew input; cmdMsg input; vref output; wref output
function [vref, wref] = ReadCMD(IsNew, cmdMsg)
persistent vref0 wref0
if isempty(vref0)
    vref0=0;
    wref0=0;
end
if IsNew
    vref0=cmdMsg.Linear.X;
    wref0=cmdMsg.Angular.Z;
end
vref=vref0;wref=wref0;

== matlab function b6_pfc_rl/Subsystem/Car Pose Listener1/Subsystem/sensor2vCar ==
  data: x_init output; y_init output; yaw_init output; flag output; poseNew input; poseMsg input
function [x_init,y_init,yaw_init,flag] = sensor2vCar(poseNew, poseMsg)
persistent x0 y0 yaw0 yaw1 x0_init y0_init yaw0_init fStart
if isempty(x0)
    x0=-10; y0=-10; yaw0=0; yaw1=0;   
    x0_init=-10;y0_init=-10;yaw0_init=0;
    fStart=0;
end
if poseNew
    if x0==poseMsg.Pose.Pose.Position.X&&y0==poseMsg.Pose.Pose.Position.Y
        flag=1;
    else
        x0=poseMsg.Pose.Pose.Position.X;
        y0=poseMsg.Pose.Pose.Position.Y;   
        %yaw2=atan2(2*(poseMsg.Pose.Pose.Orientation.Z*poseMsg.Pose.Pose.Orientation.W),1-2*(poseMsg.Pose.Pose.Orientation.Z^2)); 
        eul=quat2eul([poseMsg.Pose.Pose.Orientation.W,poseMsg.Pose.Pose.Orientation.X,poseMsg.Pose.Pose.Orientation.Y,poseMsg.Pose.Pose.Orientation.Z]);
        yaw2=eul(1);
        %对前后角度差使用积分，恢复yaw的连续性
        yaw0=yaw0+angdiff(yaw1,yaw2);
        yaw1=yaw2;
        flag=0;        
        x0_init=x0;
        y0_init=y0;
        yaw0_init=yaw0;
        fStart=1;
    end 
else
    if fStart
        flag=1;
    else
        flag=0;
    end
end

x_init=x0_init;y_init=y0_init;yaw_init=yaw0_init;

== matlab function b6_pfc_rl/controller/MATLAB Function4 ==
  data: z output; pos1 input
function z = plot_a_square(pos1)
% 
% persistent Waypoints idx
% if isempty(Waypoints)
%     Waypoints=[0.2,0.2;1.8 0.2;1.8 1.8;0.2 1.8];
%     idx=0;
% end
% if idx==0
%     %初始化
%     [~,idx]=max([norm(Waypoints(1,:)-pos1(1:2)'),norm(Waypoints(2,:)-pos1(1:2)'),norm(Waypoints(3,:)-pos1(1:2)'),norm(Waypoints(4,:)-pos1(1:2)')]);
% end
% 
% if norm([Waypoints(idx,:)-pos1(1:2)'])<0.25
%     idx=idx+1;
%     if idx>length(Waypoints(:,1))
%         idx=1;
%     end
% end
% z=Waypoints(idx,:);


persistent Waypoints idx

if isempty(Waypoints)
    Waypoints=[0.5,0.5;1.5 0.5;1.5 1.5;0.5 1.5];
    idx=2;
end

if idx == 4
    pre_waypt = Waypoints(4-1,:)';
    curr_waypt = Waypoints(idx,:)';
    next_waypt = Waypoints(1,:)';
else
    if idx == 1
        pre_waypt = Waypoints(4,:)';
        curr_waypt = Waypoints(1,:)';
        next_waypt = Waypoints(2,:)';
    else
        pre_waypt = Waypoints(idx-1,:)';
        curr_waypt = Waypoints(idx,:)';
        next_waypt = Waypoints(idx+1,:)';
    end
end

pre_q = vec_norm(curr_waypt, pre_waypt);
next_q = vec_norm(next_waypt, curr_waypt);

curr_n = vec_normalize(pre_q + next_q);
curr_diff = vec_norm(pos1(1:2), curr_waypt);

flag = dot(curr_diff, curr_n);

if flag >=0

    if idx < 4
        idx = idx + 1;
    else
        idx = 1;
    end
end

idx
z=Waypoints(idx,:)

end

function result = vec_normalize(vec)
    mag = vec_mag(vec);

    if mag>0
        result = vec * (1.0/mag);
    else
        result = [0.0, 0.0];
    end
end

function result = vec_norm(vec1, vec2)
    result = vec1 - vec2;
    result = vec_normalize(result);
end

function result = vec_mag(vec)
    result = sqrt(vec(1)*vec(1)+ vec(2)*vec(2));
end

== matlab function b6_pfc_rl/controller/Ego Car 4/Signal Process ==
  data: observation output size=[1 9]; obs_flag output; pose1 input; pose2 input; leader_linear_vel input size=1; ego_linear_vel input size=1; ego_omega_vel input size=1; last_ego_omega_vel input
function [observation, obs_flag] = ...
    car2(pose1,pose2,leader_linear_vel, ego_linear_vel, ego_omega_vel, last_ego_omega_vel)


persistent sim_step  yaw_delta lateral_rel_dist

if isempty(sim_step)
    sim_step = 0;
end

if isempty(yaw_delta)
    yaw_delta = 0.0;
end

if isempty(lateral_rel_dist)
    lateral_rel_dist = 0.0;
end

x1=pose1(1);
y1=pose1(2);
yaw1=pose1(3);

x2=pose2(1);
y2=pose2(2);
yaw2=pose2(3);
obs_flag = 1;
observation = zeros(1,9);

if isnan(yaw1)||isnan(yaw2)
    observation = zeros(1,9);
    obs_flag = 0;
    yaw_delta_new = 0.0;
    lateral_rel_dist_new = 0.0;
else
    yaw_delta_new = angdiff(yaw1, yaw2);
    
    [~, lateral_rel_dist_new, longitudinal_rel_dist_new] = heng_zong_dist_calc(x1,y1,x2,y2, yaw1);
    
    observation = get_obs(x1,x2,y1,y2,lateral_rel_dist_new, longitudinal_rel_dist_new, ...
        yaw_delta_new, leader_linear_vel, ego_linear_vel, yaw_delta, lateral_rel_dist); 
end

sim_step = sim_step + 1;
yaw_delta = yaw_delta_new;
lateral_rel_dist = lateral_rel_dist_new;

end

function [rel_dist, heng_dist, zong_dist] = heng_zong_dist_calc(x1,y1,x2,y2, yaw1)

rel_yaw = atan2(y2-y1, x2-x1);

yaw_delta = angdiff(yaw1, rel_yaw);

rel_dist = sqrt(power(x2-x1,2.0)+power(y2-y1,2.0));

heng_dist = rel_dist*sin(yaw_delta);

zong_dist = rel_dist*cos(yaw_delta);

end

function v_ref = get_ref_velocity(leader_linear_vel, ego_linear_vel, longitudinal_rel_dist)
    t_gap = 1.0;
    D_default = 0.3;
    ego_v_set = 0.2;
    d_safe = ego_linear_vel * t_gap + D_default;

    if d_safe > longitudinal_rel_dist
        v_ref = min(leader_linear_vel, ego_v_set);
    else
        v_ref = ego_v_set;
    end
end

function observation = get_obs(x1,x2,y1,y2,lateral_rel_dist_new, longitudinal_rel_dist_new, ...
    yaw_delta_new, leader_linear_vel, ego_linear_vel, yaw_delta, lateral_rel_dist)  
    % 状态空间
    % longitudinal_rel_dist 前车与后车的纵向相对距离
    % lateral_rel_dist 前车与后车的横向相对距离
    % yaw_delta 前车与后车的航向角偏差
    % ego_linear_vel 后车的线速度
    % e_v 后车的参考速度与线速度之差
    % lateral_rel_dist_dot 前车与后车的横向相对距离变化率
    % yaw_delta_dot 前车与后车的航向角偏差变化率

    % 计算前车与后车的相对位置
    x_delta = x1 - x2;
    y_delta = y1 - y2;
    
    % 计算后车的横向偏移距离变化率和相对航向角变化率
    lateral_rel_dist_dot = lateral_rel_dist_new - lateral_rel_dist;
    yaw_delta_dot = yaw_delta_new - yaw_delta;

    % 计算后车的参考速度与线速度之差
    v_ref = get_ref_velocity(leader_linear_vel, ego_linear_vel, longitudinal_rel_dist_new);
    e_v = v_ref - ego_linear_vel;

    observation = [x_delta/2.0, y_delta/2.0, longitudinal_rel_dist_new/2.0, e_v/0.5, ego_linear_vel/0.5, ...
        lateral_rel_dist_new/2.0, lateral_rel_dist_dot/2.0, yaw_delta_new/pi, yaw_delta_dot/pi];
end

function flag = EnvisDone(rel_dist, lateral_rel_dist, longitudinal_rel_dist)
    flag = 0;
    avoid_dist = 0.14;

    max_lateral_rel_dist= 0.45;
    min_longitudinal_rel_dist = -0.5;

    if rel_dist <= avoid_dist
        flag = 1;
    end

    if longitudinal_rel_dist <= min_longitudinal_rel_dist
        flag = 1;
    end
    
    if abs(lateral_rel_dist) >= max_lateral_rel_dist
        flag = 1;
    end
end

function reward = reward_calc(e_v, lateral_rel_dist, ego_linear_vel, ego_omega_vel, last_ego_omega_vel, isDone, sim_step)
    F_t = 0.0;
    M_t = 0.0;
    H_t = 0.0;
    delta_omega = 0.0;
    
    e_v_square = e_v * e_v;
    lateral_rel_dist_square = lateral_rel_dist * lateral_rel_dist;

    if isDone==1
        F_t = 1.0;
    end

    if e_v_square < 1.0
        M_t = 1.0;
    end

    if lateral_rel_dist_square<0.01
        H_t = 1.0;
    end

    if sim_step >= 2
        delta_omega = ego_omega_vel - last_ego_omega_vel;
    end

    reward = -0.1*e_v_square - 0.1*ego_linear_vel*ego_linear_vel -0.1*lateral_rel_dist_square ...
         - 0.5*ego_omega_vel*ego_omega_vel -0.4*delta_omega*delta_omega - 10.0*F_t + M_t + + 2.0*H_t;

end

== matlab function b6_pfc_rl/Subsystem/Car Pose Listener/Subsystem/sensor2vCar4 ==
  data: V output; W output; VW_New input; VW_Msg input
function [V,W] = sensor2vCar(VW_New, VW_Msg)
persistent v0 w0
if isempty(v0)
    v0=0; 
    w0=0;    
end
if VW_New
    v0=VW_Msg.Linear.X;
    w0=VW_Msg.Angular.Z;
end

V=v0;
W=-w0;

== matlab function b6_pfc_rl/ROS_simulation/ros2/MATLAB Function3 ==
  data: IsNew input; cmdMsg input; vref output; wref output
function [vref, wref] = ReadCMD(IsNew, cmdMsg)
persistent vref0 wref0
if isempty(vref0)
    vref0=0;
    wref0=0;
end
if IsNew
    vref0=cmdMsg.Linear.X;
    wref0=cmdMsg.Angular.Z;
end
vref=vref0;wref=wref0;

== matlab function b6_pfc_rl/ROS_simulation/ros3/MATLAB Function3 ==
  data: IsNew input; cmdMsg input; vref output; wref output
function [vref, wref] = ReadCMD(IsNew, cmdMsg)
persistent vref0 wref0
if isempty(vref0)
    vref0=0;
    wref0=0;
end
if IsNew
    vref0=cmdMsg.Linear.X;
    wref0=cmdMsg.Angular.Z;
end
vref=vref0;wref=wref0;

== matlab function b6_pfc_rl/ROS_simulation/ros4/MATLAB Function3 ==
  data: IsNew input; cmdMsg input; vref output; wref output
function [vref, wref] = ReadCMD(IsNew, cmdMsg)
persistent vref0 wref0
if isempty(vref0)
    vref0=0;
    wref0=0;
end
if IsNew
    vref0=cmdMsg.Linear.X;
    wref0=cmdMsg.Angular.Z;
end
vref=vref0;wref=wref0;

== matlab function b6_pfc_rl/controller/MATLAB Function2 ==
  settings: updateMethod=DISCRETE
  data: obs input double size=9; pose2 input; action output double size=[1,2]; obs_flag input
function action = one_car_pfc(obs, pose2, obs_flag)

longitudinal_rel_dist = obs(3);
lateral_rel_dist = obs(6);

if longitudinal_rel_dist > -0.25 && abs(lateral_rel_dist) <=0.225 && longitudinal_rel_dist < 0
    action = double(PFC_Policy(obs));
else
    action = simple_pfc(obs(1), obs(2), pose2(3));
end

if obs_flag==0
    action = [0.0, 0.0];
end

end

function action = simple_pfc(x_delta, y_delta, yaw2)
    kk = -1.0;

    new_theta_cmd = atan2(y_delta, x_delta);
    
    delta_theta = angdiff(yaw2, new_theta_cmd);

    angular_speed = kk * delta_theta;
     
    new_omega_cmd = angular_speed;

    action = [0.225, new_omega_cmd];

end

== matlab function b6_pfc_rl/controller/Ego Car 1/Signal Process ==
  data: observation output size=[1,9]; obs_flag output; pose1 input; pose2 input; leader_linear_vel input size=1; ego_linear_vel input size=1; ego_omega_vel input size=1; last_ego_omega_vel input
function [observation, obs_flag] = ...
    car2(pose1,pose2,leader_linear_vel, ego_linear_vel, ego_omega_vel, last_ego_omega_vel)


persistent sim_step  yaw_delta lateral_rel_dist

if isempty(sim_step)
    sim_step = 0;
end

if isempty(yaw_delta)
    yaw_delta = 0.0;
end

if isempty(lateral_rel_dist)
    lateral_rel_dist = 0.0;
end

x1=pose1(1);
y1=pose1(2);
yaw1=pose1(3);

x2=pose2(1);
y2=pose2(2);
yaw2=pose2(3);
obs_flag = 1;
observation = zeros(1,9);

if isnan(yaw1)||isnan(yaw2)
    observation = zeros(1,9);
    obs_flag = 0;
    yaw_delta_new = 0.0;
    lateral_rel_dist_new = 0.0;
else
    yaw_delta_new = angdiff(yaw1, yaw2);
    
    [~, lateral_rel_dist_new, longitudinal_rel_dist_new] = heng_zong_dist_calc(x1,y1,x2,y2, yaw1);
    
    observation = get_obs(x1,x2,y1,y2,lateral_rel_dist_new, longitudinal_rel_dist_new, ...
        yaw_delta_new, leader_linear_vel, ego_linear_vel, yaw_delta, lateral_rel_dist); 
end

sim_step = sim_step + 1;
yaw_delta = yaw_delta_new;
lateral_rel_dist = lateral_rel_dist_new;

end

function [rel_dist, heng_dist, zong_dist] = heng_zong_dist_calc(x1,y1,x2,y2, yaw1)

rel_yaw = atan2(y2-y1, x2-x1);

yaw_delta = angdiff(yaw1, rel_yaw);

rel_dist = sqrt(power(x2-x1,2.0)+power(y2-y1,2.0));

heng_dist = rel_dist*sin(yaw_delta);

zong_dist = rel_dist*cos(yaw_delta);

end

function v_ref = get_ref_velocity(leader_linear_vel, ego_linear_vel, longitudinal_rel_dist)
    t_gap = 1.0;
    D_default = 0.3;
    ego_v_set = 0.2;
    d_safe = ego_linear_vel * t_gap + D_default;

    if d_safe > longitudinal_rel_dist
        v_ref = min(leader_linear_vel, ego_v_set);
    else
        v_ref = ego_v_set;
    end
end

function observation = get_obs(x1,x2,y1,y2,lateral_rel_dist_new, longitudinal_rel_dist_new, ...
    yaw_delta_new, leader_linear_vel, ego_linear_vel, yaw_delta, lateral_rel_dist)  
    % 状态空间
    % longitudinal_rel_dist 前车与后车的纵向相对距离
    % lateral_rel_dist 前车与后车的横向相对距离
    % yaw_delta 前车与后车的航向角偏差
    % ego_linear_vel 后车的线速度
    % e_v 后车的参考速度与线速度之差
    % lateral_rel_dist_dot 前车与后车的横向相对距离变化率
    % yaw_delta_dot 前车与后车的航向角偏差变化率

    % 计算前车与后车的相对位置
    x_delta = x1 - x2;
    y_delta = y1 - y2;
    
    % 计算后车的横向偏移距离变化率和相对航向角变化率
    lateral_rel_dist_dot = lateral_rel_dist_new - lateral_rel_dist;
    yaw_delta_dot = yaw_delta_new - yaw_delta;

    % 计算后车的参考速度与线速度之差
    v_ref = get_ref_velocity(leader_linear_vel, ego_linear_vel, longitudinal_rel_dist_new);
    e_v = v_ref - ego_linear_vel;

    observation = [x_delta/2.0, y_delta/2.0, longitudinal_rel_dist_new/2.0, e_v/0.5, ego_linear_vel/0.5, ...
        lateral_rel_dist_new/2.0, lateral_rel_dist_dot/2.0, yaw_delta_new/pi, yaw_delta_dot/pi];
end

function flag = EnvisDone(rel_dist, lateral_rel_dist, longitudinal_rel_dist)
    flag = 0;
    avoid_dist = 0.14;

    max_lateral_rel_dist= 0.45;
    min_longitudinal_rel_dist = -0.5;

    if rel_dist <= avoid_dist
        flag = 1;
    end

    if longitudinal_rel_dist <= min_longitudinal_rel_dist
        flag = 1;
    end
    
    if abs(lateral_rel_dist) >= max_lateral_rel_dist
        flag = 1;
    end
end

function reward = reward_calc(e_v, lateral_rel_dist, ego_linear_vel, ego_omega_vel, last_ego_omega_vel, isDone, sim_step)
    F_t = 0.0;
    M_t = 0.0;
    H_t = 0.0;
    delta_omega = 0.0;
    
    e_v_square = e_v * e_v;
    lateral_rel_dist_square = lateral_rel_dist * lateral_rel_dist;

    if isDone==1
        F_t = 1.0;
    end

    if e_v_square < 1.0
        M_t = 1.0;
    end

    if lateral_rel_dist_square<0.01
        H_t = 1.0;
    end

    if sim_step >= 2
        delta_omega = ego_omega_vel - last_ego_omega_vel;
    end

    reward = -0.1*e_v_square - 0.1*ego_linear_vel*ego_linear_vel -0.1*lateral_rel_dist_square ...
         - 0.5*ego_omega_vel*ego_omega_vel -0.4*delta_omega*delta_omega - 10.0*F_t + M_t + + 2.0*H_t;

end
